simulink library "csc_tlt_takeoff_landing_table_guidance_mtv_lib"  (R2014b)
settings: Solver=ode45  StartTime=0.0  StopTime=10.0  RelTol=1e-3
values from neighbouring files (symbols this model uses):
  fsw_dt = 0.1    [csc_est_state_estimation_test.m]    (also in csci_fsw_mtv_init.m)
  init_int_egc = .3    (= 0.3)    [csu_waypoint_hover_guidance_init.m]
  kd_acs = 5.03    [csu_waypoint_hover_guidance_init.m]
  kd_egc = 1    [csu_waypoint_hover_guidance_init.m]
  ki_acs = 0    [csu_waypoint_hover_guidance_init.m]
  ki_egc = 1    [csu_waypoint_hover_guidance_init.m]
  kp_acs = 6.32    [csu_waypoint_hover_guidance_init.m]
  kp_egc = 1    [csu_waypoint_hover_guidance_init.m]
  tlt_waypoint_hover_translate_table = [ 4      2       6       0.00        0.00        1.60        3.0;       3      3       6       0.00        0.00        0.0         1e12;       ]    [csu_waypoint_hover_guidance_init.m]
undefined symbols (not defined in the file or in its folder): tlt_waypoint_hover_translate_table_length
libraries: simulink x3, util_extra_lib x3, util_info_lib x1, util_common_lib x1
settings Model: Creator=escrane  LastModifiedBy=tgorton

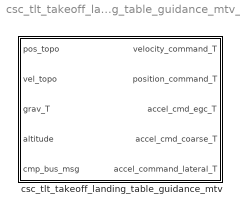
== system csc_tlt_takeoff_landing_table_guidance_mtv_lib ==
  csc_tlt_takeoff_landing_table_guidance_mtv : Subsystem  VariantControl=tlt_altitude_takeoff_table

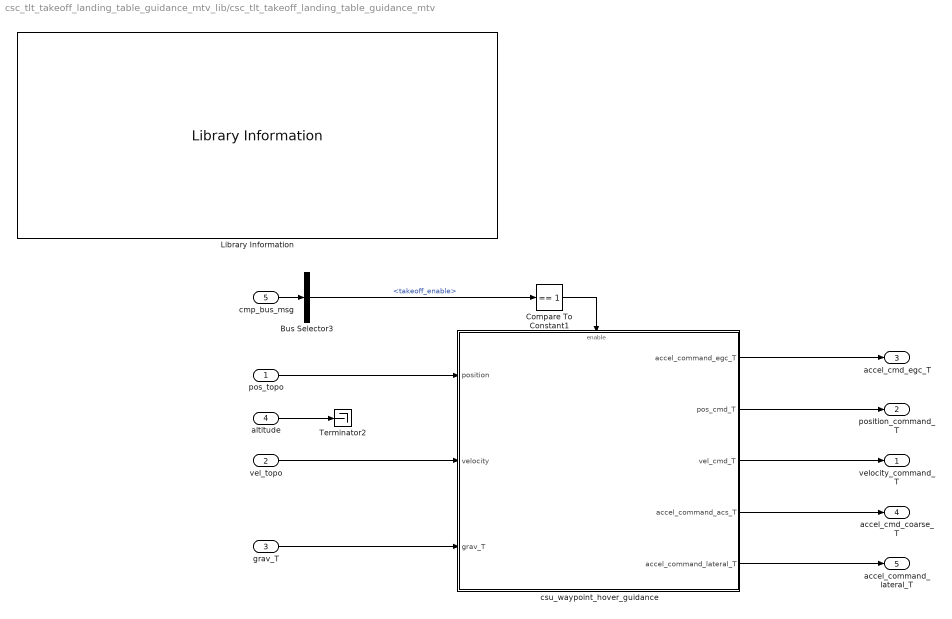
== system csc_tlt_takeoff_landing_table_guidance_mtv_lib/csc_tlt_takeoff_landing_table_guidance_mtv ==
  pos_topo : Inport
  vel_topo : Inport  Port=2
  grav_T : Inport  Port=3
  altitude : Inport  Port=4
  cmp_bus_msg : Inport  Port=5
  Bus Selector3 : BusSelector  OutputSignals=takeoff_enable
  Compare To Constant1 : simulink/Logic and Bit Operations/Compare To Constant  relop===  const=1  OutDataTypeStr=boolean
  Library Information : util_info_lib/Library Information  owner='NONE'
  Terminator2 : Terminator
  csu_waypoint_hover_guidance : Subsystem  TreatAsAtomicUnit=on
  velocity_command_T : Outport
  position_command_T : Outport  Port=2
  accel_cmd_egc_T : Outport  Port=3
  accel_cmd_coarse_T : Outport  Port=4
  accel_command_lateral_T : Outport  Port=5
  wires:
  Compare To Constant1/1 -> csu_waypoint_hover_guidance/Enable
  csu_waypoint_hover_guidance/5(accel_command_lateral_T) -> accel_command_lateral_T/1
  altitude/1 -> Terminator2/1
  csu_waypoint_hover_guidance/4(accel_command_acs_T) -> accel_cmd_coarse_T/1
  csu_waypoint_hover_guidance/1(accel_command_egc_T) -> accel_cmd_egc_T/1
  csu_waypoint_hover_guidance/2(pos_cmd_T) -> position_command_T/1
  csu_waypoint_hover_guidance/3(vel_cmd_T) -> velocity_command_T/1
  pos_topo/1 -> csu_waypoint_hover_guidance/1(position)
  Bus Selector3/1 -> Compare To Constant1/1  "<takeoff_enable>"
  grav_T/1 -> csu_waypoint_hover_guidance/3(grav_T)
  vel_topo/1 -> csu_waypoint_hover_guidance/2(velocity)
  cmp_bus_msg/1 -> Bus Selector3/1

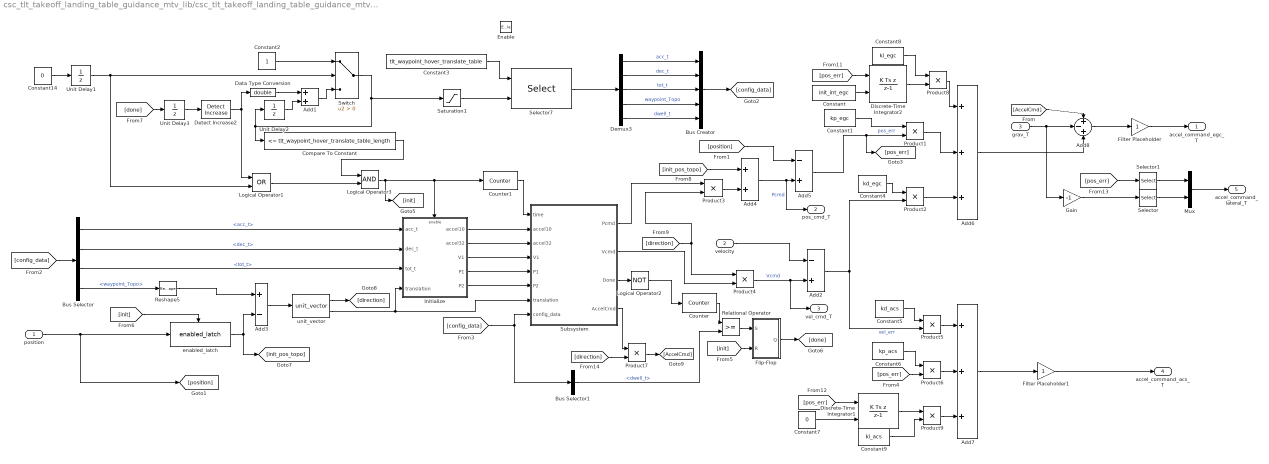
== system csc_tlt_takeoff_landing_table_guidance_mtv_lib/csc_tlt_takeoff_landing_table_guidance_mtv/csu_waypoint_hover_guidance ==
  position : Inport
  velocity : Inport  Port=2
  grav_T : Inport  Port=3
  Enable : EnablePort  StatesWhenEnabling=reset
  Add1 : Sum  InputSameDT=on
  Add2 : Sum  Inputs=-+
  Add3 : Sum  Inputs=+-
  Add4 : Sum
  Add5 : Sum  Inputs=-+
  Add6 : Sum  Inputs=+++
  Add7 : Sum  Inputs=+++
  Add8 : Sum  Inputs=+-+  InputSameDT=on
  Bus Creator : BusCreator  Inputs=5
  Bus Selector : BusSelector  OutputSignals=acc_t,dec_t,tot_t,waypoint_Topo
  Bus Selector1 : BusSelector  OutputSignals=dwell_t
  Compare To Constant : simulink/Logic and Bit Operations/Compare To Constant  relop=<=  const=tlt_waypoint_hover_translate_table_length  OutDataTypeStr=boolean
  Constant : Constant  Value=init_int_egc
  Constant1 : Constant  Value=kp_egc
  Constant14 : Constant  Value=0
  Constant2 : Constant
  Constant3 : Constant  Value=tlt_waypoint_hover_translate_table
  Constant4 : Constant  Value=kd_egc
  Constant5 : Constant  Value=kd_acs
  Constant6 : Constant  Value=kp_acs
  Constant7 : Constant  Value=0
  Constant8 : Constant  Value=ki_egc
  Constant9 : Constant  Value=ki_acs
  Counter : util_extra_lib/Counter  dt=fsw_dt  v0=0  dv=fsw_dt
  Counter1 : util_extra_lib/Counter  dt=fsw_dt  v0=0  dv=fsw_dt
  Data Type Conversion : DataTypeConversion  OutDataTypeStr=double
  Demux3 : Demux  Outputs=[1 1 1 3 1]
  Detect Increase2 : simulink/Logic and Bit Operations/Detect Increase  vinit=0.0  InputProcessing=Inherited  OutDataTypeStr=boolean
  Discrete-Time Integrator1 : DiscreteIntegrator  IntegratorMethod=Integration: Backward Euler  gainval=1  InitialConditionSource=external  InitialConditionSetting=State (most efficient)  SampleTime=fsw_dt  LimitOutput=on  UpperSaturationLimit=1e6  LowerSaturationLimit=-1e6
  Discrete-Time Integrator2 : DiscreteIntegrator  IntegratorMethod=Integration: Backward Euler  gainval=1  InitialConditionSource=external  InitialConditionSetting=State (most efficient)  SampleTime=fsw_dt  LimitOutput=on  UpperSaturationLimit=1e6  LowerSaturationLimit=-1e6
  Filter Placeholder : Gain
  Filter Placeholder1 : Gain
  Flip-Flop : Subsystem  mask(SRFlipFlop){initial_condition=0}
      mask prompts: initial_condition "Initial condition (state of Q):"
  Gain : Gain  Gain=-1
  Initialize : Subsystem  TreatAsAtomicUnit=on
  Logical Operator1 : Logic  Operator=OR  AllPortsSameDT=off  OutDataTypeStr=boolean
  Logical Operator2 : Logic  Operator=NOT  AllPortsSameDT=off  OutDataTypeStr=boolean
  Logical Operator3 : Logic  AllPortsSameDT=off  OutDataTypeStr=boolean
  Mux : Mux  Inputs=[2 1]
  Product{1..9} (9 alike) : Product
  Relational Operator : RelationalOperator  OutDataTypeStr=boolean
  Reshape5 : Reshape  OutputDimensionality=Column vector (2-D)
  Saturation1 : Saturate  UpperLimit=tlt_waypoint_hover_translate_table_length  LowerLimit=1
  Selector : Selector  InputPortWidth=3  Indices=[3]
  Selector1 : Selector  InputPortWidth=3  Indices=[1 2]
  Selector7 : Selector  NumberOfDimensions=2  InputPortWidth=3  IndexOptions=Index vector (port),Select all  Indices=[1 3],1  OutputSizes=1,1
  Subsystem : Subsystem
  Switch : Switch  Criteria=u2 > Threshold
  Unit Delay1 : UnitDelay  InitialCondition=1  SampleTime=-1
  Unit Delay2 : UnitDelay  SampleTime=-1
  Unit Delay3 : UnitDelay  SampleTime=-1
  enabled_latch : util_common_lib/enabled_latch  initial_output=0
  unit_vector : util_extra_lib/unit_vector  SystemSampleTime=-1
  accel_command_egc_T : Outport
  pos_cmd_T : Outport  Port=2
  vel_cmd_T : Outport  Port=3
  accel_command_acs_T : Outport  Port=4
  accel_command_lateral_T : Outport  Port=5  InitialOutput=[0 0 1]'
  wires:
  Mux/1 -> accel_command_lateral_T/1
  Selector/1 -> Mux/2
  Selector1/1 -> Mux/1
  Gain/1 -> Selector/1
  [pos_err] -> Selector1/1
  [pos_err] -> Discrete-Time Integrator2/1
  Unit Delay1/1 -> Switch/2, Logical Operator1/2
  Constant14/1 -> Unit Delay1/1
  Discrete-Time Integrator2/1 -> Product8/2
  Product8/1 -> Add6/1
  Discrete-Time Integrator1/1 -> Product9/1
  Product9/1 -> Add7/3
  Constant9/1 -> Product9/2
  Constant8/1 -> Product8/1
  [direction] -> Product7/2
  Product7/1 -> [AccelCmd]
  grav_T/1 -> Gain/1, Add8/2
  [AccelCmd] -> Add8/1
  Logical Operator3/1 -> [init], Initialize/Enable, Counter1/1
  Filter Placeholder1/1 -> accel_command_acs_T/1
  Filter Placeholder/1 -> accel_command_egc_T/1
  Add8/1 -> Filter Placeholder/1
  Subsystem/4(AccelCmd) -> Product7/1
  Constant7/1 -> Discrete-Time Integrator1/2
  [pos_err] -> Discrete-Time Integrator1/1
  Constant/1 -> Discrete-Time Integrator2/2
  Constant6/1 -> Product6/1
  Constant5/1 -> Product5/1
  [pos_err] -> Product6/2
  Product6/1 -> Add7/2
  Product5/1 -> Add7/1
  Add7/1 -> Filter Placeholder1/1
  Compare To Constant/1 -> Logical Operator3/1
  Add6/1 -> Add8/3
  Product2/1 -> Add6/3
  Product1/1 -> Add6/2
  Constant4/1 -> Product2/1
  Add2/1 -> Product2/2, Product5/2  "vel_err"
  Constant1/1 -> Product1/1
  Add5/1 -> Product1/2, [pos_err]  "pos_err"
  [position] -> Add5/1
  velocity/1 -> Add2/1
  Saturation1/1 -> Selector7/2
  Data Type Conversion/1 -> Add1/1
  Product4/1 -> Add2/2, vel_cmd_T/1  "Vcmd"
  Subsystem/2(Vcmd) -> Product4/2
  [direction] -> Product4/1, Product3/2
  Subsystem/1(Pcmd) -> Product3/1
  Product3/1 -> Add4/2
  unit_vector/1 -> [direction]
  Add4/1 -> Add5/2, pos_cmd_T/1  "Pcmd"
  [init_pos_topo] -> Add4/1
  Unit Delay3/1 -> Detect Increase2/1
  [done] -> Unit Delay3/1
  Flip-Flop/1(Q) -> [done]
  Relational Operator/1 -> Flip-Flop/1(S)
  [init] -> Flip-Flop/2(R)
  Counter/1 -> Relational Operator/1
  Reshape5/1 -> Add3/1
  enabled_latch/1 -> Add3/2, [init_pos_topo]
  [init] -> enabled_latch/Enable
  Bus Selector1/1 -> Relational Operator/2  "<dwell_t>"
  Counter1/1 -> Subsystem/1(time)
  Logical Operator2/1 -> Counter/1
  [config_data] -> Bus Selector1/1, Subsystem/8(config_data)
  Subsystem/3(Done) -> Logical Operator2/1
  Initialize/5(P2) -> Subsystem/6(P2)
  Initialize/4(P1) -> Subsystem/5(P1)
  Initialize/3(V1) -> Subsystem/4(V1)
  Initialize/2(accel32) -> Subsystem/3(accel32)
  Initialize/1(accel10) -> Subsystem/2(accel10)
  Bus Selector/2 -> Initialize/2(dec_t)  "<dec_t>"
  Bus Selector/1 -> Initialize/1(acc_t)  "<acc_t>"
  Bus Selector/3 -> Initialize/3(tot_t)  "<tot_t>"
  Bus Creator/1 -> [config_data]
  Demux3/4 -> Bus Creator/4  "waypoint_Topo"
  Demux3/5 -> Bus Creator/5  "dwell_t"
  Demux3/3 -> Bus Creator/3  "tot_t"
  Demux3/2 -> Bus Creator/2  "dec_t"
  Demux3/1 -> Bus Creator/1  "acc_t"
  Selector7/1 -> Demux3/1
  unit_vector/2 -> Initialize/4(translation), Subsystem/7(translation)
  Add3/1 -> unit_vector/1
  position/1 -> enabled_latch/1, [position]
  Bus Selector/4 -> Reshape5/1  "<waypoint_Topo>"
  Logical Operator1/1 -> Logical Operator3/2
  [config_data] -> Bus Selector/1
  Constant3/1 -> Selector7/1
  Detect Increase2/1 -> Data Type Conversion/1, Logical Operator1/1
  Add1/1 -> Switch/3
  Constant2/1 -> Switch/1
  Unit Delay2/1 -> Add1/2
  Switch/1 -> Saturation1/1, Compare To Constant/1, Unit Delay2/1

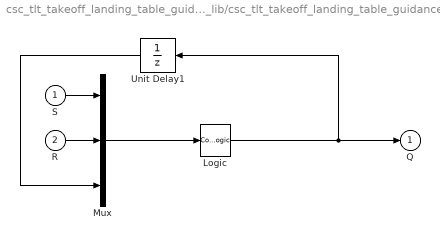
== system csc_tlt_takeoff_landing_table_guidance_mtv_lib/csc_tlt_takeoff_landing_table_guidance_mtv/csu_waypoint_hover_guidance/Flip-Flop ==
  S : Inport
  R : Inport  Port=2
  Logic : CombinatorialLogic  TruthTable=[0; 1; 0; 0; 1; 1; 1; 0]
  Mux : Mux  Inputs=3
  Unit Delay1 : UnitDelay  InitialCondition=initial_condition  SampleTime=-1
  Q : Outport  InitialOutput=0
  wires:
  Mux/1 -> Logic/1
  Logic/1 -> Unit Delay1/1, Q/1
  S/1 -> Mux/1
  R/1 -> Mux/2
  Unit Delay1/1 -> Mux/3

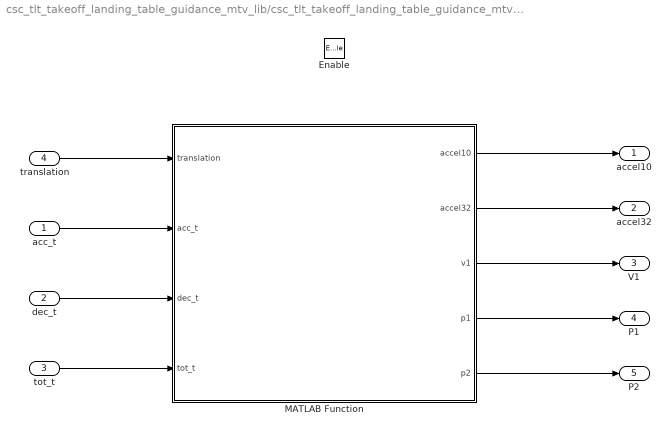
== system csc_tlt_takeoff_landing_table_guidance_mtv_lib/csc_tlt_takeoff_landing_table_guidance_mtv/csu_waypoint_hover_guidance/Initialize ==
  acc_t : Inport
  dec_t : Inport  Port=2
  tot_t : Inport  Port=3
  translation : Inport  Port=4
  Enable : EnablePort
  MATLAB Function : MATLAB Function  TreatAsAtomicUnit=on
  accel10 : Outport
  accel32 : Outport  Port=2
  V1 : Outport  Port=3
  P1 : Outport  Port=4
  P2 : Outport  Port=5
  wires:
  MATLAB Function/5(p2) -> P2/1
  MATLAB Function/4(p1) -> P1/1
  MATLAB Function/3(v1) -> V1/1
  MATLAB Function/2(accel32) -> accel32/1
  MATLAB Function/1(accel10) -> accel10/1
  tot_t/1 -> MATLAB Function/4(tot_t)
  dec_t/1 -> MATLAB Function/3(dec_t)
  acc_t/1 -> MATLAB Function/2(acc_t)
  translation/1 -> MATLAB Function/1(translation)

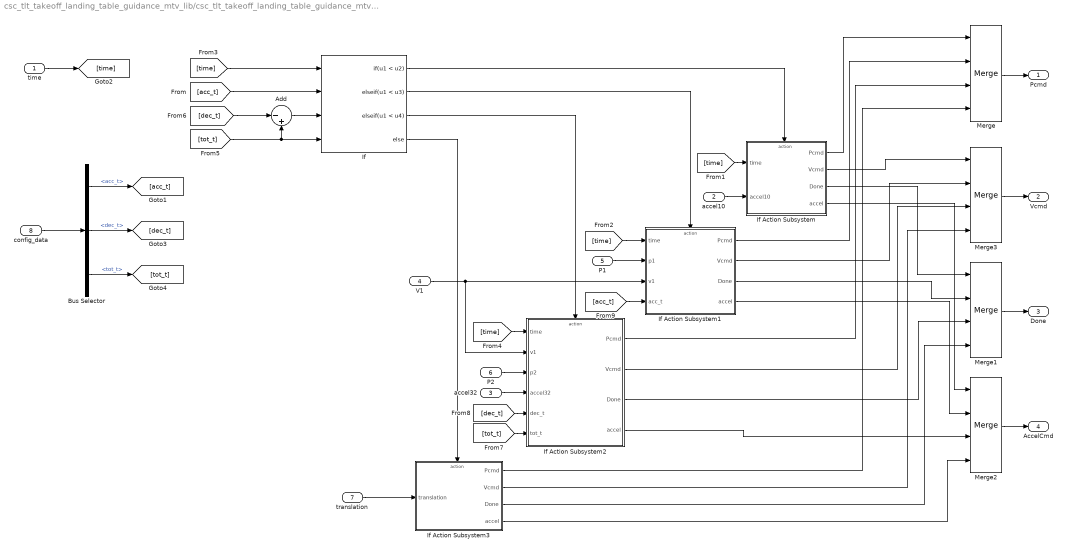
== system csc_tlt_takeoff_landing_table_guidance_mtv_lib/csc_tlt_takeoff_landing_table_guidance_mtv/csu_waypoint_hover_guidance/Subsystem ==
  time : Inport
  accel10 : Inport  Port=2
  accel32 : Inport  Port=3
  V1 : Inport  Port=4
  P1 : Inport  Port=5
  P2 : Inport  Port=6
  translation : Inport  Port=7
  config_data : Inport  Port=8
  Add : Sum  Inputs=|-+
  Bus Selector : BusSelector  OutputSignals=acc_t,dec_t,tot_t
  If : If  NumInputs=4  IfExpression=u1 < u2  ElseIfExpressions=u1 < u3,u1 < u4
  If Action Subsystem : Subsystem  TreatAsAtomicUnit=on
  If Action Subsystem1 : Subsystem  TreatAsAtomicUnit=on
  If Action Subsystem2 : Subsystem  TreatAsAtomicUnit=on
  If Action Subsystem3 : Subsystem  TreatAsAtomicUnit=on
  Merge{,1..3} (4 alike) : Merge  Inputs=4
  Pcmd : Outport
  Vcmd : Outport  Port=2
  Done : Outport  Port=3
  AccelCmd : Outport  Port=4
  wires:
  Merge2/1 -> AccelCmd/1
  If Action Subsystem3/4(accel) -> Merge2/4
  If Action Subsystem2/4(accel) -> Merge2/3
  If Action Subsystem1/4(accel) -> Merge2/2
  If Action Subsystem/4(accel) -> Merge2/1
  [acc_t] -> If Action Subsystem1/4(acc_t)
  translation/1 -> If Action Subsystem3/1(translation)
  P2/1 -> If Action Subsystem2/3(p2)
  P1/1 -> If Action Subsystem1/2(p1)
  V1/1 -> If Action Subsystem1/3(v1), If Action Subsystem2/2(v1)
  accel32/1 -> If Action Subsystem2/4(accel32)
  accel10/1 -> If Action Subsystem/2(accel10)
  [dec_t] -> If Action Subsystem2/5(dec_t)
  [tot_t] -> If Action Subsystem2/6(tot_t)
  [dec_t] -> Add/1
  Add/1 -> If/3
  [tot_t] -> If/4, Add/2
  [acc_t] -> If/2
  Merge1/1 -> Done/1
  If Action Subsystem3/3(Done) -> Merge1/4
  If Action Subsystem2/3(Done) -> Merge1/3
  If Action Subsystem1/3(Done) -> Merge1/2
  If Action Subsystem/3(Done) -> Merge1/1
  If Action Subsystem3/2(Vcmd) -> Merge3/4
  If Action Subsystem2/2(Vcmd) -> Merge3/3
  If Action Subsystem1/2(Vcmd) -> Merge3/2
  If Action Subsystem/2(Vcmd) -> Merge3/1
  Merge3/1 -> Vcmd/1
  If Action Subsystem3/1(Pcmd) -> Merge/4
  If Action Subsystem2/1(Pcmd) -> Merge/3
  If Action Subsystem1/1(Pcmd) -> Merge/2
  Merge/1 -> Pcmd/1
  If Action Subsystem/1(Pcmd) -> Merge/1
  If/4 -> If Action Subsystem3/Action
  [time] -> If Action Subsystem2/1(time)
  If/3 -> If Action Subsystem2/Action
  [time] -> If Action Subsystem1/1(time)
  If/2 -> If Action Subsystem1/Action
  If/1 -> If Action Subsystem/Action
  [time] -> If Action Subsystem/1(time)
  [time] -> If/1
  Bus Selector/3 -> [tot_t]  "<tot_t>"
  Bus Selector/2 -> [dec_t]  "<dec_t>"
  Bus Selector/1 -> [acc_t]  "<acc_t>"
  config_data/1 -> Bus Selector/1
  time/1 -> [time]

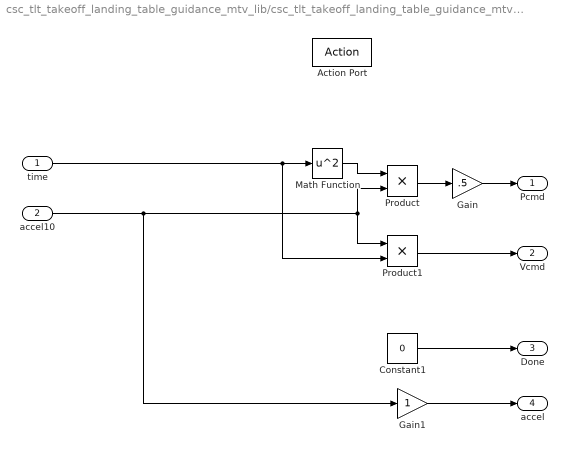
== system csc_tlt_takeoff_landing_table_guidance_mtv_lib/csc_tlt_takeoff_landing_table_guidance_mtv/csu_waypoint_hover_guidance/Subsystem/If Action Subsystem ==
  time : Inport
  accel10 : Inport  Port=2
  Action Port : ActionPort
  Constant1 : Constant  Value=0
  Gain : Gain  Gain=.5
  Gain1 : Gain
  Math Function : Math  Operator=square  SaturateOnIntegerOverflow=on
  Product : Product  RndMeth=Zero
  Product1 : Product  RndMeth=Zero
  Pcmd : Outport
  Vcmd : Outport  Port=2
  Done : Outport  Port=3  InitialOutput=1
  accel : Outport  Port=4  InitialOutput=1
  wires:
  Gain1/1 -> accel/1
  Constant1/1 -> Done/1
  Product1/1 -> Vcmd/1
  Gain/1 -> Pcmd/1
  Product/1 -> Gain/1
  accel10/1 -> Product1/1, Product/2, Gain1/1
  Math Function/1 -> Product/1
  time/1 -> Product1/2, Math Function/1

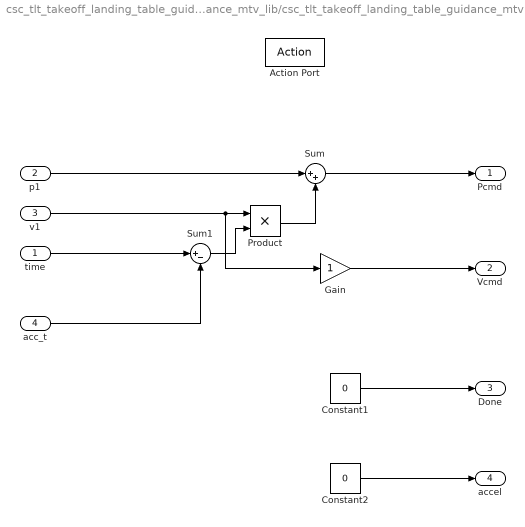
== system csc_tlt_takeoff_landing_table_guidance_mtv_lib/csc_tlt_takeoff_landing_table_guidance_mtv/csu_waypoint_hover_guidance/Subsystem/If Action Subsystem1 ==
  time : Inport
  p1 : Inport  Port=2
  v1 : Inport  Port=3
  acc_t : Inport  Port=4
  Action Port : ActionPort
  Constant1 : Constant  Value=0
  Constant2 : Constant  Value=0
  Gain : Gain
  Product : Product  RndMeth=Zero
  Sum : Sum  Inputs=|++
  Sum1 : Sum  Inputs=|+-
  Pcmd : Outport
  Vcmd : Outport  Port=2
  Done : Outport  Port=3  InitialOutput=1
  accel : Outport  Port=4  InitialOutput=1
  wires:
  Constant2/1 -> accel/1
  Constant1/1 -> Done/1
  Gain/1 -> Vcmd/1
  acc_t/1 -> Sum1/2
  Product/1 -> Sum/2
  Sum1/1 -> Product/2
  v1/1 -> Gain/1, Product/1
  time/1 -> Sum1/1
  p1/1 -> Sum/1
  Sum/1 -> Pcmd/1

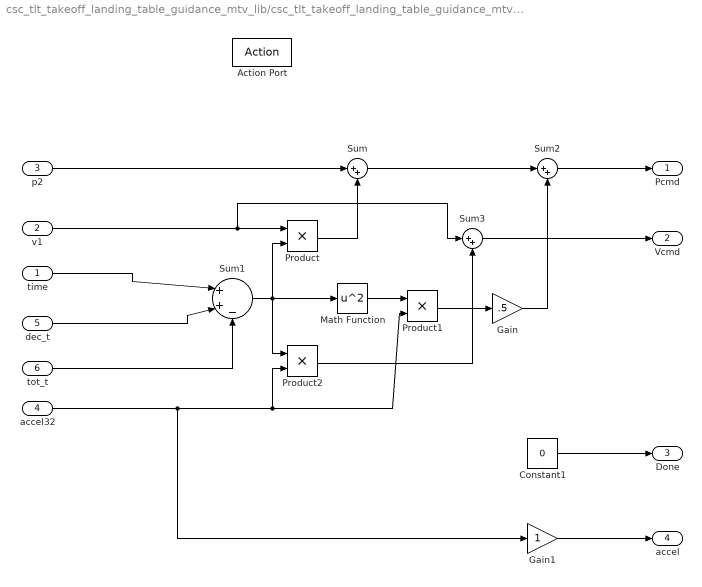
== system csc_tlt_takeoff_landing_table_guidance_mtv_lib/csc_tlt_takeoff_landing_table_guidance_mtv/csu_waypoint_hover_guidance/Subsystem/If Action Subsystem2 ==
  time : Inport
  v1 : Inport  Port=2
  p2 : Inport  Port=3
  accel32 : Inport  Port=4
  dec_t : Inport  Port=5
  tot_t : Inport  Port=6
  Action Port : ActionPort
  Constant1 : Constant  Value=0
  Gain : Gain  Gain=.5
  Gain1 : Gain
  Math Function : Math  Operator=square  SaturateOnIntegerOverflow=on
  Product : Product  RndMeth=Zero
  Product1 : Product  RndMeth=Zero
  Product2 : Product  RndMeth=Zero
  Sum : Sum  Inputs=|++
  Sum1 : Sum  Inputs=|++-
  Sum2 : Sum  Inputs=|++
  Sum3 : Sum  Inputs=|++
  Pcmd : Outport
  Vcmd : Outport  Port=2
  Done : Outport  Port=3  InitialOutput=1
  accel : Outport  Port=4  InitialOutput=1
  wires:
  Gain1/1 -> accel/1
  Constant1/1 -> Done/1
  tot_t/1 -> Sum1/3
  dec_t/1 -> Sum1/2
  Sum3/1 -> Vcmd/1
  Product2/1 -> Sum3/2
  Sum2/1 -> Pcmd/1
  Gain/1 -> Sum2/2
  Sum/1 -> Sum2/1
  Product1/1 -> Gain/1
  accel32/1 -> Product1/2, Product2/2, Gain1/1
  Math Function/1 -> Product1/1
  Product/1 -> Sum/2
  p2/1 -> Sum/1
  v1/1 -> Sum3/1, Product/1
  Sum1/1 -> Product2/1, Math Function/1, Product/2
  time/1 -> Sum1/1

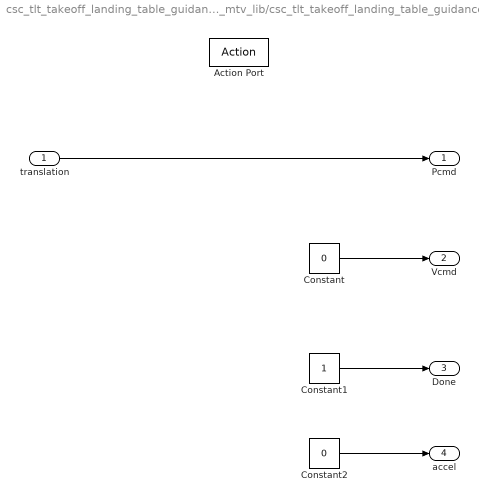
== system csc_tlt_takeoff_landing_table_guidance_mtv_lib/csc_tlt_takeoff_landing_table_guidance_mtv/csu_waypoint_hover_guidance/Subsystem/If Action Subsystem3 ==
  translation : Inport
  Action Port : ActionPort
  Constant : Constant  Value=0
  Constant1 : Constant
  Constant2 : Constant  Value=0
  Pcmd : Outport
  Vcmd : Outport  Port=2
  Done : Outport  Port=3  InitialOutput=1
  accel : Outport  Port=4  InitialOutput=1
  wires:
  Constant2/1 -> accel/1
  Constant1/1 -> Done/1
  Constant/1 -> Vcmd/1
  translation/1 -> Pcmd/1

== matlab function csc_tlt_takeoff_landing_table_guidance_mtv_lib/csc_tlt_takeoff_landing_table_guidance_mtv/csu_waypoint_hover_guidance/Initialize/MATLAB Function ==
  data: translation input; accel10 output; acc_t input; dec_t input; tot_t input; accel32 output; v1 output; p1 output; p2 output
function [accel10,accel32,v1,p1,p2] = calculate_params(translation,acc_t,dec_t,tot_t)
%#codegen

y = 2*translation;
temp_den = 2*tot_t-acc_t-dec_t;
if abs(temp_den) >1e-10
    v1 = y/temp_den;
else
    v1 = 0;
end
if abs(acc_t) > 1e-10
    accel10 = v1/acc_t;
else
    accel10 = 0;
end
if abs(dec_t) > 1e-10
    accel32 = -v1/dec_t;
else
    accel32 = 0;
end
p1 = v1*acc_t/2;
p2 = translation - v1*dec_t/2;
